simulink model "fuzzyControllerTestBench"  (R2013b)
settings: Solver=FixedStepDiscrete  StartTime=0.0  StopTime=4  RelTol=1e-3
libraries: fuzblock x6
settings Model: NumberOfSteps=1000  Creator=Raj  LastModifiedBy=Rajpaged
settings OptimizationCC: UseIntDivNetSlope=on  UseFloatMulNetSlope=on  EfficientMapNaN2IntZero=off  OptimizeModelRefInitCode=on  LifeSpan=1  MaxStackSize=64
settings DebuggingCC: ConsistencyChecking=warning  TimeAdjustmentMsg=warning  StateNameClashWarn=warning
settings HardwareCC: ProdLargestAtomicInteger=Long  ProdLargestAtomicFloat=Double  ProdEndianess=LittleEndian  ProdHWDeviceType=ARM Compatible->ARM Cortex
settings RTWCC: SystemTargetFile=ert.tlc  GenCodeOnly=on  TemplateMakefile=ert_default_tmf  Description=Embedded Coder  ProcessScript=ert_make_rtw_hook
settings CodeAppCC: IgnoreCustomStorageClasses=off
settings ERTTargetCC: CodeReplacementLibrary=C89/C90 (ANSI)  IncludeMdlTerminateFcn=off  SuppressErrorStatus=on  SupportNonFinite=off  ERTCustomFileTemplate=example_file_process.tlc  ERTFilePackagingFormat=CompactWithDataFile  ConvertIfToSwitch=on

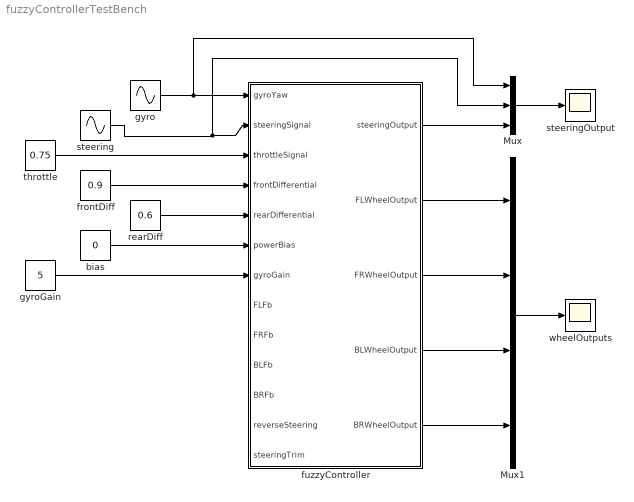
== system fuzzyControllerTestBench ==
  Mux : Mux  Inputs=3
  Mux1 : Mux
  bias : Constant  Value=0
  frontDiff : Constant  Value=0.9
  fuzzyController : Subsystem
  gyro : Sin  Frequency=20  SampleTime=0
  gyroGain : Constant  Value=5
  rearDiff : Constant  Value=0.6
  steering : Sin  Frequency=8  SampleTime=0
  steeringOutput : Scope
  throttle : Constant  Value=0.75
  wheelOutputs : Scope
      settings: YMin=0.575  YMax=0.825
  wires:
  frontDiff/1 -> fuzzyController/4(frontDifferential)
  rearDiff/1 -> fuzzyController/5(rearDifferential)
  bias/1 -> fuzzyController/6(powerBias)
  fuzzyController/5(BRWheelOutput) -> Mux1/4
  Mux/1 -> steeringOutput/1
  fuzzyController/4(BLWheelOutput) -> Mux1/3
  fuzzyController/3(FRWheelOutput) -> Mux1/2
  Mux1/1 -> wheelOutputs/1
  steering/1 -> Mux/2, fuzzyController/2(steeringSignal)
  fuzzyController/2(FLWheelOutput) -> Mux1/1
  fuzzyController/1(steeringOutput) -> Mux/3
  gyro/1 -> fuzzyController/1(gyroYaw), Mux/1
  throttle/1 -> fuzzyController/3(throttleSignal)
  gyroGain/1 -> fuzzyController/7(gyroGain)

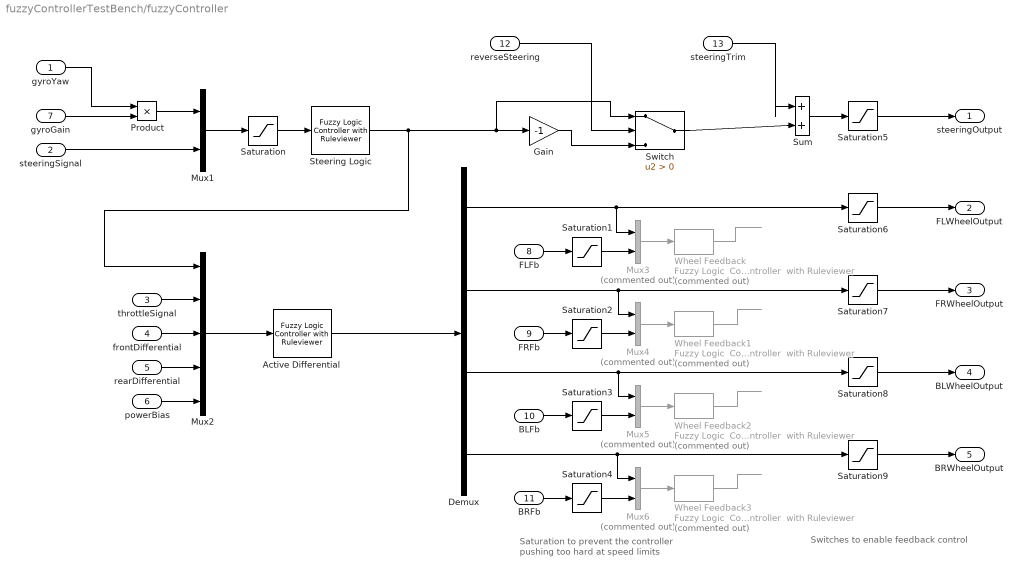
== system fuzzyControllerTestBench/fuzzyController ==
  note: Saturation to prevent the controller
      | pushing too hard at speed limits
  note: Switches to enable feedback control
  gyroYaw : Inport  OutDataTypeStr=double
  steeringSignal : Inport  Port=2  OutDataTypeStr=double
  throttleSignal : Inport  Port=3  OutDataTypeStr=double
  frontDifferential : Inport  Port=4  OutDataTypeStr=double
  rearDifferential : Inport  Port=5  OutDataTypeStr=double
  powerBias : Inport  Port=6  OutDataTypeStr=double
  gyroGain : Inport  Port=7  OutDataTypeStr=double
  FLFb : Inport  Port=8  OutDataTypeStr=double
  FRFb : Inport  Port=9  OutDataTypeStr=double
  BLFb : Inport  Port=10  OutDataTypeStr=double
  BRFb : Inport  Port=11  OutDataTypeStr=double
  reverseSteering : Inport  Port=12  OutDataTypeStr=double
  steeringTrim : Inport  Port=13  OutDataTypeStr=double
  Active Differential : fuzblock/Fuzzy Logic  Controller  with Ruleviewer  fismatrix=activeDifferential  Ts=0.01
  Demux : Demux
  Gain : Gain  Gain=-1
  Mux1 : Mux  Inputs=2
  Mux2 : Mux  Inputs=5
  Mux{3..6} (4 alike) : Mux  Commented=on  Inputs=2
  Product : Product
  Saturation{,5..9} (6 alike) : Saturate  UpperLimit=1  LowerLimit=-1
  Saturation{1..4} (4 alike) : Saturate  UpperLimit=1  LowerLimit=0
  Steering Logic : fuzblock/Fuzzy Logic  Controller  with Ruleviewer  fismatrix=steeringModule  Ts=0.01
  Sum : Sum  Inputs=|++
  Switch : Switch  Criteria=u2 > Threshold
  Wheel Feedback{,1..3} (4 alike) : fuzblock/Fuzzy Logic  Controller  with Ruleviewer  Commented=on  fismatrix=steeringModule  Ts=0.01
  steeringOutput : Outport  OutDataTypeStr=double
  FLWheelOutput : Outport  Port=2  OutDataTypeStr=double
  FRWheelOutput : Outport  Port=3  OutDataTypeStr=double
  BLWheelOutput : Outport  Port=4  OutDataTypeStr=double
  BRWheelOutput : Outport  Port=5  OutDataTypeStr=double
  wires:
  Mux2/1 -> Active Differential/1
  Active Differential/1 -> Demux/1
  steeringSignal/1 -> Mux1/2
  throttleSignal/1 -> Mux2/2
  powerBias/1 -> Mux2/5
  rearDifferential/1 -> Mux2/4
  frontDifferential/1 -> Mux2/3
  Product/1 -> Mux1/1
  gyroYaw/1 -> Product/1
  gyroGain/1 -> Product/2
  Wheel Feedback/1 -> ?
  Mux3/1 -> Wheel Feedback/1
  Demux/1 -> Saturation6/1, Mux3/1
  Mux6/1 -> Wheel Feedback3/1
  Wheel Feedback2/1 -> ?
  Wheel Feedback1/1 -> ?
  Mux4/1 -> Wheel Feedback1/1
  FLFb/1 -> Saturation1/1
  BRFb/1 -> Saturation4/1
  BLFb/1 -> Saturation3/1
  FRFb/1 -> Saturation2/1
  Wheel Feedback3/1 -> ?
  Demux/4 -> Saturation9/1, Mux6/1
  Demux/3 -> Saturation8/1, Mux5/1
  Demux/2 -> Saturation7/1, Mux4/1
  Mux5/1 -> Wheel Feedback2/1
  Saturation1/1 -> Mux3/2
  Saturation2/1 -> Mux4/2
  Saturation3/1 -> Mux5/2
  Saturation4/1 -> Mux6/2
  Steering Logic/1 -> Mux2/1, Switch/1, Gain/1
  Saturation/1 -> Steering Logic/1
  Mux1/1 -> Saturation/1
  Gain/1 -> Switch/3
  reverseSteering/1 -> Switch/2
  Switch/1 -> Sum/2
  steeringTrim/1 -> Sum/1
  Saturation5/1 -> steeringOutput/1
  Saturation6/1 -> FLWheelOutput/1
  Saturation7/1 -> FRWheelOutput/1
  Saturation8/1 -> BLWheelOutput/1
  Saturation9/1 -> BRWheelOutput/1
  Sum/1 -> Saturation5/1
